simulink model "FlyByWire"  (R2020b)
settings: Solver=FixedStepAuto  StartTime=0.0  StopTime=10.0  FixedStep=0.02  RelTol=1e-3
InitFcn:
  | run('fbw_data_init_fbw_output.m')
values from neighbouring files (symbols this model uses):
  fbw_output_MATLABStruct = struct    [fbw_data_init_fbw_output.m]
undefined symbols (not defined in the file or in its folder): pitch, roll, sim
libraries: fbw_library x19, simulink_extras x13, simulink x2
settings Model: DataDictionary=fbw_data.sldd  Creator=Andreas  LastModifiedBy=Andreas

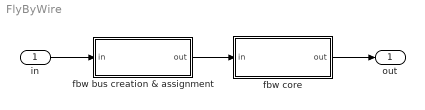
== system FlyByWire ==
  in : Inport  OutDataTypeStr=Bus: fbw_input
  fbw bus creation & assignment : Subsystem
  fbw core : Subsystem
  out : Outport  OutDataTypeStr=Bus: fbw_output
  wires:
  fbw core/1(out) -> out/1
  in/1 -> fbw bus creation & assignment/1(in)
  fbw bus creation & assignment/1(out) -> fbw core/1(in)

== system FlyByWire/fbw bus creation & assignment ==
  in : Inport
  Bus Assignment : BusAssignment  AssignedSignals=sim.raw.time,sim.raw.data,sim.raw.input
  Bus Selector : BusSelector  OutputSignals=time,data,input
  Constant : Constant  Value=fbw_output_MATLABStruct  OutDataTypeStr=Bus: fbw_output
  out : Outport
  wires:
  Constant/1 -> Bus Assignment/1
  in/1 -> Bus Selector/1
  Bus Assignment/1 -> out/1
  Bus Selector/2 -> Bus Assignment/3  "<data>"
  Bus Selector/3 -> Bus Assignment/4  "<input>"
  Bus Selector/1 -> Bus Assignment/2  "<time>"

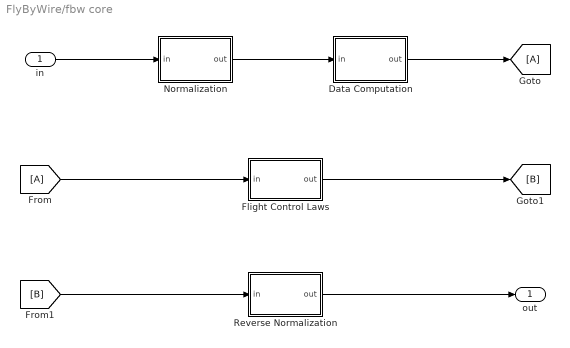
== system FlyByWire/fbw core ==
  in : Inport
  Data Computation : Subsystem
  Flight Control Laws : Subsystem
  Normalization : Subsystem
  Reverse Normalization : Subsystem
  out : Outport
  wires:
  Normalization/1(out) -> Data Computation/1(in)
  [B] -> Reverse Normalization/1(in)
  Data Computation/1(out) -> [A]
  [A] -> Flight Control Laws/1(in)
  in/1 -> Normalization/1(in)
  Reverse Normalization/1(out) -> out/1
  Flight Control Laws/1(out) -> [B]

== system FlyByWire/fbw core/Data Computation ==
  In Bus Element2 : Inport  PortName=in
  In Bus Element1 : Inport  PortName=in
  Bus Assignment : BusAssignment  AssignedSignals=sim.data_computed
  Calculation : Subsystem
  out : Outport
  wires:
  In Bus Element2/1 -> Calculation/1(in)
  In Bus Element1/1 -> Bus Assignment/1
  Bus Assignment/1 -> out/1
  Calculation/1(out) -> Bus Assignment/2

== system FlyByWire/fbw core/Flight Control Laws ==
  In Bus Element3 : Inport  PortName=in
  In Bus Element1 : Inport  PortName=in
  In Bus Element2 : Inport  PortName=in
  Bus Assignment : BusAssignment  AssignedSignals=pitch,roll
  Bus Selector : BusSelector  OutputSignals=roll
  Bus Selector1 : BusSelector  OutputSignals=pitch
  Pitch : Subsystem
  Roll : Subsystem
  out : Outport
  wires:
  Bus Selector1/1 -> Bus Assignment/2  "<pitch>"
  Roll/1(out) -> Bus Selector/1
  In Bus Element1/1 -> Bus Assignment/1
  Bus Selector/1 -> Bus Assignment/3  "<roll>"
  In Bus Element2/1 -> Roll/1(in)
  In Bus Element3/1 -> Pitch/1(in)
  Bus Assignment/1 -> out/1
  Pitch/1(Output) -> Bus Selector1/1

== system FlyByWire/fbw core/Normalization ==
  In Bus Element2 : Inport  PortName=in
  In Bus Element : Inport  PortName=in  Element=sim.raw.data
  In Bus Element1 : Inport  PortName=in  Element=sim.raw.input
  In Bus Element3 : Inport  PortName=in  Element=sim.raw.time
  Bus Assignment : BusAssignment  AssignedSignals=sim.time,sim.data,sim.input
  normalize data : Subsystem
  normalize input : Subsystem
  time : Subsystem
  out : Outport
  wires:
  In Bus Element2/1 -> Bus Assignment/1
  Bus Assignment/1 -> out/1
  In Bus Element/1 -> normalize data/1(in)
  normalize data/1(out) -> Bus Assignment/3
  In Bus Element1/1 -> normalize input/1(in)
  normalize input/1(out) -> Bus Assignment/4
  In Bus Element3/1 -> time/1(in)
  time/1(out) -> Bus Assignment/2

== system FlyByWire/fbw core/Reverse Normalization ==
  In Bus Element9 : Inport  PortName=in
  In Bus Element1 : Inport  PortName=in
  Bus Assignment : BusAssignment  AssignedSignals=sim.raw.output
  Subsystem : Subsystem
  out : Outport
  wires:
  In Bus Element9/1 -> Bus Assignment/1
  Bus Assignment/1 -> out/1
  In Bus Element1/1 -> Subsystem/1(in)
  Subsystem/1(out) -> Bus Assignment/2

== system FlyByWire/fbw core/Data Computation/Calculation ==
  In Bus Element1 : Inport  PortName=in  Element=sim.data.gear_strut_compression_1
  In Bus Element2 : Inport  PortName=in  Element=sim.data.gear_strut_compression_2
  Chart : Stateflow chart  TreatAsAtomicUnit=on
  Out Bus Element : Outport  PortName=out  Element=on_ground
  wires:
  Chart/1(on_ground) -> Out Bus Element/1
  In Bus Element1/1 -> Chart/1(gear_strut_compression_1)
  In Bus Element2/1 -> Chart/2(gear_strut_compression_2)

== system FlyByWire/fbw core/Flight Control Laws/Pitch ==
  in : Inport
  Automatic Trim : Subsystem
  pitch : Subsystem
  pitch:computed : Subsystem
  pitch:integrated : Subsystem
  pitch:output : Subsystem
  pitch:vote : Subsystem
  Output : Outport
  wires:
  Automatic Trim/1(out) -> Output/1
  [A] -> Automatic Trim/1(in)
  pitch:output/1(out) -> [A]
  pitch:integrated/1(out) -> pitch:output/1(in)
  pitch:vote/1(out) -> pitch:integrated/1(in)
  pitch/1(out) -> pitch:vote/1(in)
  in/1 -> pitch:computed/1(in)
  pitch:computed/1(out) -> pitch/1(in)

== system FlyByWire/fbw core/Flight Control Laws/Roll ==
  in : Inport
  roll:computed : Subsystem
  roll:normal : Subsystem
  roll:output : Subsystem
  out : Outport
  wires:
  roll:output/1(out) -> out/1
  roll:normal/1(out) -> roll:output/1(in)
  roll:computed/1(out) -> roll:normal/1(in)
  in/1 -> roll:computed/1(in)

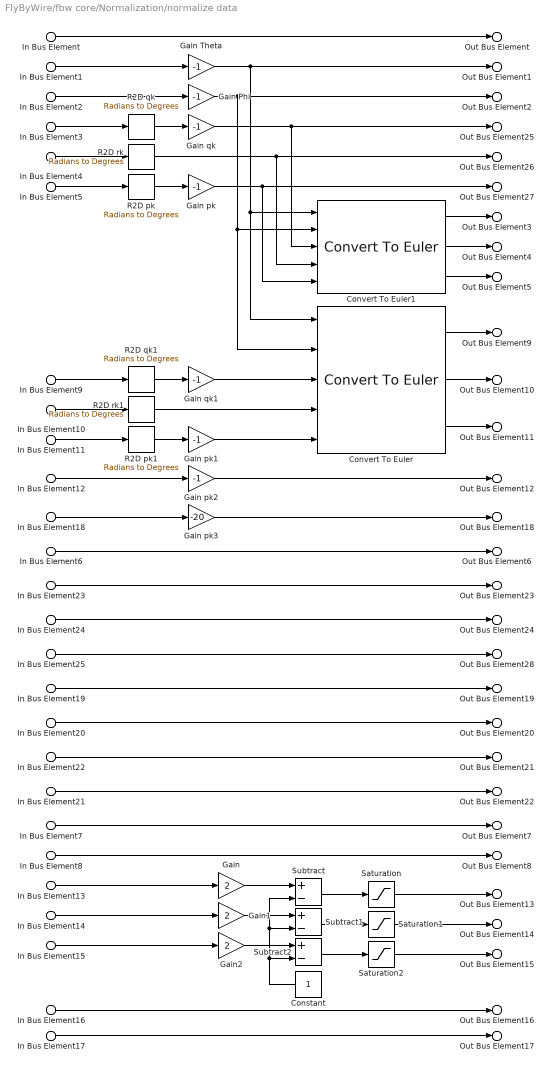
== system FlyByWire/fbw core/Normalization/normalize data ==
  In Bus Element : Inport  PortName=in  Element=nz_g
  In Bus Element1 : Inport  PortName=in  Element=Theta_deg
  In Bus Element2 : Inport  PortName=in  Element=Phi_deg
  In Bus Element3 : Inport  PortName=in  Element=q_rad_s
  In Bus Element4 : Inport  PortName=in  Element=r_rad_s
  In Bus Element5 : Inport  PortName=in  Element=p_rad_s
  In Bus Element6 : Inport  PortName=in  Element=V_ias_kn
  In Bus Element7 : Inport  PortName=in  Element=H_radio_ft
  In Bus Element8 : Inport  PortName=in  Element=CG_percent_MAC
  In Bus Element9 : Inport  PortName=in  Element=q_dot_rad_s2
  In Bus Element10 : Inport  PortName=in  Element=r_dot_rad_s2
  In Bus Element11 : Inport  PortName=in  Element=p_dot_rad_s2
  In Bus Element12 : Inport  PortName=in  Element=eta_trim_deg
  In Bus Element13 : Inport  PortName=in  Element=gear_animation_pos_0
  In Bus Element14 : Inport  PortName=in  Element=gear_animation_pos_1
  In Bus Element15 : Inport  PortName=in  Element=gear_animation_pos_2
  In Bus Element16 : Inport  PortName=in  Element=flaps_handle_index
  In Bus Element17 : Inport  PortName=in  Element=autopilot_master_on
  In Bus Element18 : Inport  PortName=in  Element=zeta_trim_pos
  In Bus Element19 : Inport  PortName=in  Element=V_tas_kn
  In Bus Element20 : Inport  PortName=in  Element=V_mach
  In Bus Element22 : Inport  PortName=in  Element=H_ft
  In Bus Element21 : Inport  PortName=in  Element=H_ind_ft
  In Bus Element23 : Inport  PortName=in  Element=alpha_deg
  In Bus Element24 : Inport  PortName=in  Element=beta_deg
  In Bus Element25 : Inport  PortName=in  Element=beta_dot_deg_s
  Constant : Constant
  Convert To Euler : fbw_library/Convert To Euler  SystemSampleTime=-1  VariantActivationTime=update diagram  Latency=0  AutoFrameSizeCalculation=off
  Convert To Euler1 : fbw_library/Convert To Euler  SystemSampleTime=-1  VariantActivationTime=update diagram  Latency=0  AutoFrameSizeCalculation=off
  Gain : Gain  Gain=2
  Gain Phi : Gain  Gain=-1
  Gain Theta : Gain  Gain=-1
  Gain pk : Gain  Gain=-1
  Gain pk1 : Gain  Gain=-1
  Gain pk2 : Gain  Gain=-1
  Gain pk3 : Gain  Gain=-20
  Gain qk : Gain  Gain=-1
  Gain qk1 : Gain  Gain=-1
  Gain1 : Gain  Gain=2
  Gain2 : Gain  Gain=2
  R2D pk : simulink_extras/Transformations/Radians to Degrees
  R2D pk1 : simulink_extras/Transformations/Radians to Degrees
  R2D qk : simulink_extras/Transformations/Radians to Degrees
  R2D qk1 : simulink_extras/Transformations/Radians to Degrees
  R2D rk : simulink_extras/Transformations/Radians to Degrees
  R2D rk1 : simulink_extras/Transformations/Radians to Degrees
  Saturation : Saturate  UpperLimit=1  LowerLimit=0
  Saturation1 : Saturate  UpperLimit=1  LowerLimit=0
  Saturation2 : Saturate  UpperLimit=1  LowerLimit=0
  Subtract : Sum  Inputs=+-
  Subtract1 : Sum  Inputs=+-
  Subtract2 : Sum  Inputs=+-
  Out Bus Element : Outport  PortName=out  Element=nz_g
  Out Bus Element1 : Outport  PortName=out  Element=Theta_deg
  Out Bus Element2 : Outport  PortName=out  Element=Phi_deg
  Out Bus Element25 : Outport  PortName=out  Element=q_deg_s
  Out Bus Element26 : Outport  PortName=out  Element=r_deg_s
  Out Bus Element27 : Outport  PortName=out  Element=p_deg_s
  Out Bus Element3 : Outport  PortName=out  Element=qk_deg_s
  Out Bus Element4 : Outport  PortName=out  Element=rk_deg_s
  Out Bus Element5 : Outport  PortName=out  Element=pk_deg_s
  Out Bus Element9 : Outport  PortName=out  Element=qk_dot_deg_s2
  Out Bus Element10 : Outport  PortName=out  Element=rk_dot_deg_s2
  Out Bus Element11 : Outport  PortName=out  Element=pk_dot_deg_s2
  Out Bus Element12 : Outport  PortName=out  Element=eta_trim_deg
  Out Bus Element18 : Outport  PortName=out  Element=zeta_trim_deg
  Out Bus Element23 : Outport  PortName=out  Element=alpha_deg
  Out Bus Element24 : Outport  PortName=out  Element=beta_deg
  Out Bus Element28 : Outport  PortName=out  Element=beta_dot_deg_s
  Out Bus Element6 : Outport  PortName=out  Element=V_ias_kn
  Out Bus Element19 : Outport  PortName=out  Element=V_tas_kn
  Out Bus Element20 : Outport  PortName=out  Element=V_mach
  Out Bus Element21 : Outport  PortName=out  Element=H_ft
  Out Bus Element22 : Outport  PortName=out  Element=H_ind_ft
  Out Bus Element7 : Outport  PortName=out  Element=H_radio_ft
  Out Bus Element8 : Outport  PortName=out  Element=CG_percent_MAC
  Out Bus Element13 : Outport  PortName=out  Element=gear_strut_compression_0
  Out Bus Element14 : Outport  PortName=out  Element=gear_strut_compression_1
  Out Bus Element15 : Outport  PortName=out  Element=gear_strut_compression_2
  Out Bus Element16 : Outport  PortName=out  Element=flaps_handle_index
  Out Bus Element17 : Outport  PortName=out  Element=autopilot_master_on
  wires:
  R2D qk/1 -> Gain qk/1
  In Bus Element4/1 -> R2D rk/1
  Gain Phi/1 -> Out Bus Element2/1, Convert To Euler/2, Convert To Euler1/2
  Gain Theta/1 -> Out Bus Element1/1, Convert To Euler/1, Convert To Euler1/1
  In Bus Element7/1 -> Out Bus Element7/1
  In Bus Element2/1 -> Gain Phi/1
  In Bus Element8/1 -> Out Bus Element8/1
  In Bus Element/1 -> Out Bus Element/1
  R2D pk/1 -> Gain pk/1
  In Bus Element6/1 -> Out Bus Element6/1
  In Bus Element1/1 -> Gain Theta/1
  In Bus Element5/1 -> R2D pk/1
  In Bus Element3/1 -> R2D qk/1
  In Bus Element11/1 -> R2D pk1/1
  In Bus Element9/1 -> R2D qk1/1
  R2D qk1/1 -> Gain qk1/1
  R2D pk1/1 -> Gain pk1/1
  In Bus Element10/1 -> R2D rk1/1
  In Bus Element12/1 -> Gain pk2/1
  Gain pk2/1 -> Out Bus Element12/1
  Gain qk1/1 -> Convert To Euler/3
  R2D rk1/1 -> Convert To Euler/4
  Gain pk1/1 -> Convert To Euler/5
  In Bus Element13/1 -> Gain/1
  In Bus Element14/1 -> Gain1/1
  In Bus Element15/1 -> Gain2/1
  Gain/1 -> Subtract/1
  Gain1/1 -> Subtract1/1
  Gain2/1 -> Subtract2/1
  Constant/1 -> Subtract/2, Subtract1/2, Subtract2/2
  Subtract2/1 -> Saturation2/1
  Subtract1/1 -> Saturation1/1
  Subtract/1 -> Saturation/1
  Saturation/1 -> Out Bus Element13/1
  Saturation1/1 -> Out Bus Element14/1
  Saturation2/1 -> Out Bus Element15/1
  In Bus Element16/1 -> Out Bus Element16/1
  In Bus Element17/1 -> Out Bus Element17/1
  In Bus Element18/1 -> Gain pk3/1
  Gain pk3/1 -> Out Bus Element18/1
  In Bus Element19/1 -> Out Bus Element19/1
  In Bus Element20/1 -> Out Bus Element20/1
  In Bus Element22/1 -> Out Bus Element21/1
  In Bus Element21/1 -> Out Bus Element22/1
  In Bus Element23/1 -> Out Bus Element23/1
  In Bus Element24/1 -> Out Bus Element24/1
  Gain qk/1 -> Out Bus Element25/1, Convert To Euler1/3
  R2D rk/1 -> Out Bus Element26/1, Convert To Euler1/4
  Gain pk/1 -> Out Bus Element27/1, Convert To Euler1/5
  Convert To Euler/1 -> Out Bus Element9/1
  Convert To Euler/2 -> Out Bus Element10/1
  Convert To Euler/3 -> Out Bus Element11/1
  Convert To Euler1/1 -> Out Bus Element3/1
  Convert To Euler1/2 -> Out Bus Element4/1
  Convert To Euler1/3 -> Out Bus Element5/1
  In Bus Element25/1 -> Out Bus Element28/1

== system FlyByWire/fbw core/Normalization/normalize input ==
  In Bus Element : Inport  PortName=in  Element=delta_eta_pos
  In Bus Element1 : Inport  PortName=in  Element=delta_xi_pos
  In Bus Element2 : Inport  PortName=in  Element=delta_zeta_pos
  Gain eta : Gain  Gain=-1
  Gain xi : Gain  Gain=-1
  Gain xi1 : Gain  Gain=-1
  Out Bus Element : Outport  PortName=out  Element=delta_eta_pos
  Out Bus Element1 : Outport  PortName=out  Element=delta_xi_pos
  Out Bus Element2 : Outport  PortName=out  Element=delta_zeta_pos
  wires:
  In Bus Element/1 -> Gain eta/1
  Gain xi/1 -> Out Bus Element1/1
  Gain eta/1 -> Out Bus Element/1
  In Bus Element1/1 -> Gain xi/1
  In Bus Element2/1 -> Gain xi1/1
  Gain xi1/1 -> Out Bus Element2/1

== system FlyByWire/fbw core/Normalization/time ==
  In Bus Element : Inport  PortName=in  Element=dt
  Delay : Delay  DelayLength=1
  Sum : Sum  Inputs=|++
  Out Bus Element : Outport  PortName=out  Element=dt
  Out Bus Element1 : Outport  PortName=out  Element=monotonic_time
  wires:
  Sum/1 -> Delay/1, Out Bus Element1/1
  In Bus Element/1 -> Sum/1, Out Bus Element/1
  Delay/1 -> Sum/2

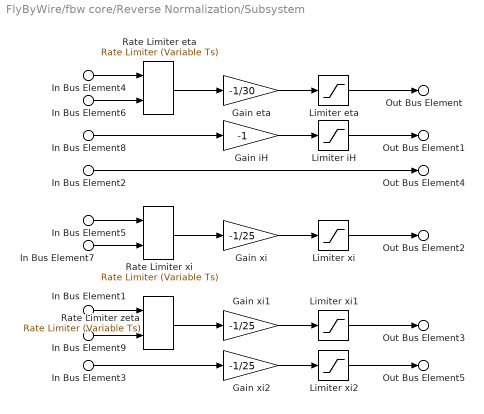
== system FlyByWire/fbw core/Reverse Normalization/Subsystem ==
  In Bus Element4 : Inport  PortName=in  Element=pitch.output.eta_deg
  In Bus Element8 : Inport  PortName=in  Element=pitch.output.eta_trim_deg
  In Bus Element2 : Inport  PortName=in  Element=pitch.data_computed.eta_trim_deg_should_write
  In Bus Element5 : Inport  PortName=in  Element=roll.output.xi_deg
  In Bus Element1 : Inport  PortName=in  Element=roll.output.zeta_deg
  In Bus Element3 : Inport  PortName=in  Element=sim.data.zeta_trim_deg
  In Bus Element6 : Inport  PortName=in  Element=sim.time.dt
  In Bus Element7 : Inport  PortName=in  Element=sim.time.dt
  In Bus Element9 : Inport  PortName=in  Element=sim.time.dt
  Gain eta : Gain  Gain=-1/30
  Gain iH : Gain  Gain=-1
  Gain xi : Gain  Gain=-1/25
  Gain xi1 : Gain  Gain=-1/25
  Gain xi2 : Gain  Gain=-1/25
  Limiter eta : Saturate  UpperLimit=1.0  LowerLimit=-1.0
  Limiter iH : Saturate  UpperLimit=13  LowerLimit=-3.5
  Limiter xi : Saturate  UpperLimit=1.0  LowerLimit=-1.0
  Limiter xi1 : Saturate  UpperLimit=1.0  LowerLimit=-1.0
  Limiter xi2 : Saturate  UpperLimit=1.0  LowerLimit=-1.0
  Rate Limiter eta : fbw_library/Rate Limiter (Variable Ts)  up=45  lo=-45  InitialCondition=0.0
  Rate Limiter xi : fbw_library/Rate Limiter (Variable Ts)  up=50  lo=-50  InitialCondition=0.0
  Rate Limiter zeta : fbw_library/Rate Limiter (Variable Ts)  up=45  lo=-45  InitialCondition=0.0
  Out Bus Element : Outport  PortName=out  Element=eta_pos
  Out Bus Element1 : Outport  PortName=out  Element=eta_trim_deg
  Out Bus Element4 : Outport  PortName=out  Element=eta_trim_deg_should_write
  Out Bus Element2 : Outport  PortName=out  Element=xi_pos
  Out Bus Element3 : Outport  PortName=out  Element=zeta_pos
  Out Bus Element5 : Outport  PortName=out  Element=zeta_trim_pos
  wires:
  Gain xi/1 -> Limiter xi/1
  Rate Limiter xi/1 -> Gain xi/1
  Rate Limiter eta/1 -> Gain eta/1
  Limiter iH/1 -> Out Bus Element1/1
  Gain eta/1 -> Limiter eta/1
  Gain iH/1 -> Limiter iH/1
  Limiter eta/1 -> Out Bus Element/1
  Limiter xi/1 -> Out Bus Element2/1
  In Bus Element4/1 -> Rate Limiter eta/1
  In Bus Element8/1 -> Gain iH/1
  In Bus Element5/1 -> Rate Limiter xi/1
  Rate Limiter zeta/1 -> Gain xi1/1
  Limiter xi1/1 -> Out Bus Element3/1
  In Bus Element1/1 -> Rate Limiter zeta/1
  Gain xi1/1 -> Limiter xi1/1
  In Bus Element2/1 -> Out Bus Element4/1
  In Bus Element3/1 -> Gain xi2/1
  Gain xi2/1 -> Limiter xi2/1
  Limiter xi2/1 -> Out Bus Element5/1
  In Bus Element6/1 -> Rate Limiter eta/2
  In Bus Element7/1 -> Rate Limiter xi/2
  In Bus Element9/1 -> Rate Limiter zeta/2

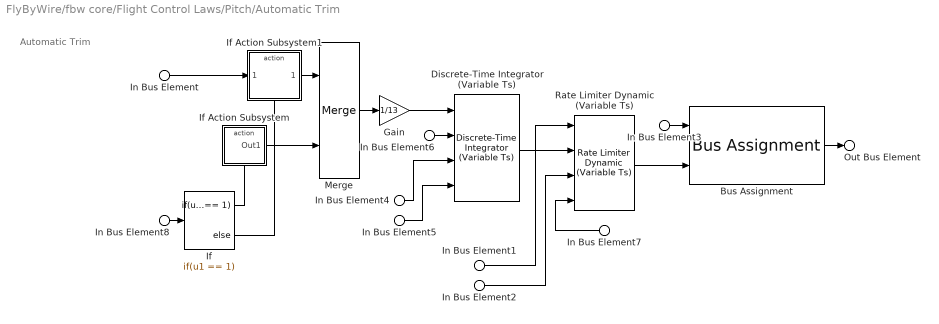
== system FlyByWire/fbw core/Flight Control Laws/Pitch/Automatic Trim ==
  note: Automatic Trim
  In Bus Element3 : Inport  PortName=in
  In Bus Element : Inport  PortName=in  Element=pitch.integrated.eta_deg
  In Bus Element8 : Inport  PortName=in  Element=pitch.data_computed.eta_trim_deg_should_freeze
  In Bus Element5 : Inport  PortName=in  Element=pitch.data_computed.eta_trim_deg_reset_deg
  In Bus Element4 : Inport  PortName=in  Element=pitch.data_computed.eta_trim_deg_reset
  In Bus Element1 : Inport  PortName=in  Element=pitch.data_computed.eta_trim_deg_rate_limit_up_deg_s
  In Bus Element2 : Inport  PortName=in  Element=pitch.data_computed.eta_trim_deg_rate_limit_lo_deg_s
  In Bus Element6 : Inport  PortName=in  Element=sim.time.dt
  In Bus Element7 : Inport  PortName=in  Element=sim.time.dt
  Bus Assignment : BusAssignment  AssignedSignals=pitch.output.eta_trim_deg
  Discrete-Time Integrator (Variable Ts) : fbw_library/Discrete-Time Integrator (Variable Ts)  Gain=1.0  ExternalReset=Level  InitialConditionSource=Input port  InitialCondition=0.0  UpperLimit=3.5  LowerLimit=-11
  Gain : Gain  Gain=1/13
  If : If  IfExpression=u1 == 1
  If Action Subsystem : Subsystem  TreatAsAtomicUnit=on
  If Action Subsystem1 : Subsystem  TreatAsAtomicUnit=on
  Merge : Merge
  Rate Limiter Dynamic (Variable Ts) : fbw_library/Rate Limiter Dynamic (Variable Ts)  InitialCondition=0.0
  Out Bus Element : Outport  PortName=out
  wires:
  In Bus Element3/1 -> Bus Assignment/1
  If Action Subsystem/1(Out1) -> Merge/2
  Discrete-Time Integrator (Variable Ts)/1 -> Rate Limiter Dynamic (Variable Ts)/2
  If Action Subsystem1/1(Out1) -> Merge/1
  Merge/1 -> Gain/1
  If/1 -> If Action Subsystem/Action
  If/2 -> If Action Subsystem1/Action
  In Bus Element/1 -> If Action Subsystem1/1(η (°))
  Bus Assignment/1 -> Out Bus Element/1
  In Bus Element1/1 -> Rate Limiter Dynamic (Variable Ts)/1
  In Bus Element2/1 -> Rate Limiter Dynamic (Variable Ts)/3
  In Bus Element5/1 -> Discrete-Time Integrator (Variable Ts)/4
  Gain/1 -> Discrete-Time Integrator (Variable Ts)/1
  Rate Limiter Dynamic (Variable Ts)/1 -> Bus Assignment/2
  In Bus Element8/1 -> If/1
  In Bus Element4/1 -> Discrete-Time Integrator (Variable Ts)/3
  In Bus Element6/1 -> Discrete-Time Integrator (Variable Ts)/2
  In Bus Element7/1 -> Rate Limiter Dynamic (Variable Ts)/4

== system FlyByWire/fbw core/Flight Control Laws/Pitch/pitch ==
  note: Pitch Laws
  In Bus Element2 : Inport  PortName=in
  In Bus Element5 : Inport  PortName=in
  Bus Assignment : BusAssignment  AssignedSignals=pitch.law_normal
  Bus Selector1 : BusSelector  OutputSignals=pitch.law_normal
  law_normal : Subsystem
  Out Bus Element3 : Outport  PortName=out
  wires:
  Bus Selector1/1 -> Bus Assignment/2  "<law_normal>"
  In Bus Element2/1 -> law_normal/1(in)
  In Bus Element5/1 -> Bus Assignment/1
  Bus Assignment/1 -> Out Bus Element3/1
  law_normal/1(out) -> Bus Selector1/1

== system FlyByWire/fbw core/Flight Control Laws/Pitch/pitch:computed ==
  In Bus Element3 : Inport  PortName=in
  In Bus Element1 : Inport  PortName=in
  Bus Assignment : BusAssignment  AssignedSignals=pitch.data_computed
  computation : Subsystem
  Out Bus Element1 : Outport  PortName=out
  wires:
  computation/1(out) -> Bus Assignment/2
  In Bus Element3/1 -> computation/1(in)
  In Bus Element1/1 -> Bus Assignment/1
  Bus Assignment/1 -> Out Bus Element1/1

== system FlyByWire/fbw core/Flight Control Laws/Pitch/pitch:integrated ==
  note: Integration
  In Bus Element : Inport  PortName=in
  In Bus Element8 : Inport  PortName=in  Element=pitch.vote.eta_dot_deg_s
  In Bus Element11 : Inport  PortName=in  Element=pitch.data_computed.in_flight
  In Bus Element9 : Inport  PortName=in  Element=pitch.data_computed.delta_eta_deg
  In Bus Element1 : Inport  PortName=in  Element=sim.time.dt
  Bus Assignment : BusAssignment  AssignedSignals=pitch.integrated.eta_deg
  Discrete-Time Integrator (Variable Ts) : fbw_library/Discrete-Time Integrator (Variable Ts)  Gain=1.0  ExternalReset=Rising  InitialConditionSource=Input port  InitialCondition=0.0  UpperLimit=17  LowerLimit=-30
  Out Bus Element : Outport  PortName=out
  wires:
  In Bus Element8/1 -> Discrete-Time Integrator (Variable Ts)/1
  In Bus Element11/1 -> Discrete-Time Integrator (Variable Ts)/3
  In Bus Element/1 -> Bus Assignment/1
  Bus Assignment/1 -> Out Bus Element/1
  Discrete-Time Integrator (Variable Ts)/1 -> Bus Assignment/2
  In Bus Element9/1 -> Discrete-Time Integrator (Variable Ts)/4
  In Bus Element1/1 -> Discrete-Time Integrator (Variable Ts)/2

== system FlyByWire/fbw core/Flight Control Laws/Pitch/pitch:output ==
  In Bus Element : Inport  PortName=in
  In Bus Element1 : Inport  PortName=in  Element=pitch.integrated.eta_deg
  In Bus Element3 : Inport  PortName=in  Element=pitch.data_computed.in_flight_gain
  In Bus Element2 : Inport  PortName=in  Element=pitch.data_computed.delta_eta_deg
  Bus Assignment : BusAssignment  AssignedSignals=pitch.output.eta_deg
  Signal Blending : fbw_library/Signal Blending  SystemSampleTime=-1  VariantActivationTime=update diagram  Latency=0  AutoFrameSizeCalculation=off
  Out Bus Element : Outport  PortName=out
  wires:
  Signal Blending/1 -> Bus Assignment/2
  In Bus Element3/1 -> Signal Blending/3
  In Bus Element1/1 -> Signal Blending/1
  In Bus Element/1 -> Bus Assignment/1
  Bus Assignment/1 -> Out Bus Element/1
  In Bus Element2/1 -> Signal Blending/2

== system FlyByWire/fbw core/Flight Control Laws/Pitch/pitch:vote ==
  note: Voting of active law
  In Bus Element1 : Inport  PortName=in
  Bus Element In : Inport  PortName=in  Element=pitch.law_normal.eta_dot_deg_s
  Bus Assignment : BusAssignment  AssignedSignals=pitch.vote.eta_dot_deg_s
  Mux : Mux  Inputs=1
  Voter : MATLAB Function  TreatAsAtomicUnit=on
  Out Bus Element1 : Outport  PortName=out
  wires:
  Bus Element In/1 -> Mux/1
  In Bus Element1/1 -> Bus Assignment/1
  Bus Assignment/1 -> Out Bus Element1/1
  Voter/1(vote) -> Bus Assignment/2
  Mux/1 -> Voter/1(input)

== system FlyByWire/fbw core/Flight Control Laws/Roll/roll:computed ==
  In Bus Element3 : Inport  PortName=in
  In Bus Element1 : Inport  PortName=in
  Bus Assignment : BusAssignment  AssignedSignals=roll.data_computed
  computation : Subsystem
  Out Bus Element1 : Outport  PortName=out
  wires:
  computation/1(out) -> Bus Assignment/2
  In Bus Element3/1 -> computation/1(in)
  In Bus Element1/1 -> Bus Assignment/1
  Bus Assignment/1 -> Out Bus Element1/1

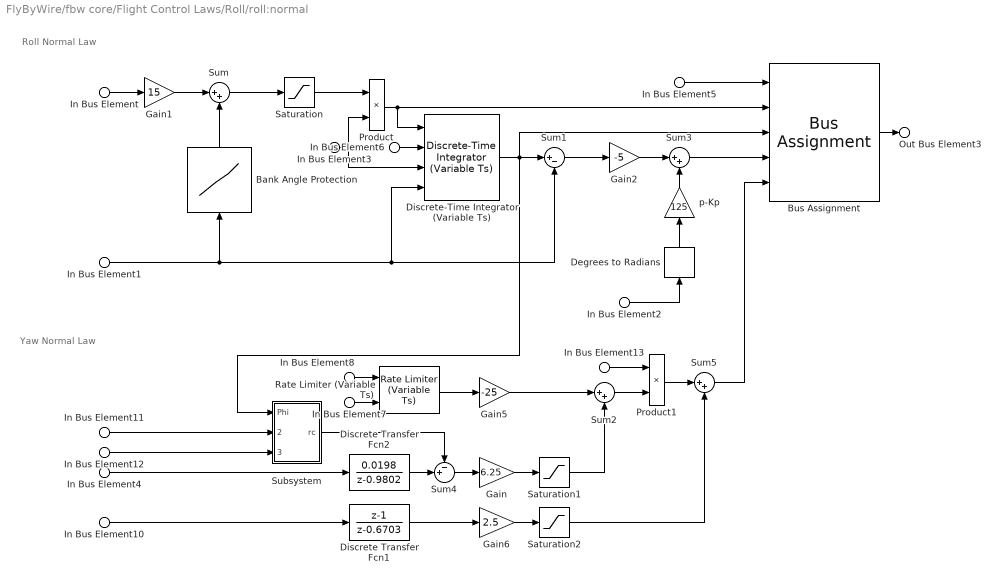
== system FlyByWire/fbw core/Flight Control Laws/Roll/roll:normal ==
  note: Yaw Normal Law
  note: Roll Normal Law
  In Bus Element5 : Inport  PortName=in
  In Bus Element : Inport  PortName=in  Element=sim.input.delta_xi_pos
  In Bus Element8 : Inport  PortName=in  Element=sim.input.delta_zeta_pos
  In Bus Element1 : Inport  PortName=in  Element=sim.data.Phi_deg
  In Bus Element2 : Inport  PortName=in  Element=sim.data.pk_deg_s
  In Bus Element10 : Inport  PortName=in  Element=sim.data.r_deg_s
  In Bus Element4 : Inport  PortName=in  Element=sim.data.r_deg_s
  In Bus Element11 : Inport  PortName=in  Element=sim.data.Theta_deg
  In Bus Element12 : Inport  PortName=in  Element=sim.data.V_tas_kn
  In Bus Element6 : Inport  PortName=in  Element=sim.time.dt
  In Bus Element7 : Inport  PortName=in  Element=sim.time.dt
  In Bus Element3 : Inport  PortName=in  Element=roll.data_computed.in_flight_gain
  In Bus Element13 : Inport  PortName=in  Element=roll.data_computed.in_flight_gain
  Bank Angle Protection : Lookup_n-D  NumberOfTableDimensions=1  BreakpointsForDimension1=[-90,-66,-33,0,33,66,90]  Table=[15,15,0,0,0,-15,-15]  InternalRulePriority=Speed  RndMeth=Simplest  InputSameDT=on
  Bus Assignment : BusAssignment  AssignedSignals=roll.law_normal.pk_c_deg_s,roll.law_normal.Phi_c_deg,roll.law_normal.xi_deg,roll.law_normal.zeta_deg
  Degrees to Radians : simulink_extras/Transformations/Degrees to Radians
  Discrete Transfer Fcn1 : DiscreteTransferFcn  Numerator=[1 -1]  Denominator=[1 -0.6703]
  Discrete Transfer Fcn2 : DiscreteTransferFcn  Numerator=[0.0198]  Denominator=[1 -0.9802]
  Discrete-Time Integrator (Variable Ts) : fbw_library/Discrete-Time Integrator (Variable Ts)  Gain=1.0  ExternalReset=Rising  InitialConditionSource=Input port  InitialCondition=0.0  UpperLimit=67  LowerLimit=-67
  Gain : Gain  Gain=6.25
  Gain1 : Gain  Gain=15
  Gain2 : Gain  Gain=-5
  Gain5 : Gain  Gain=-25
  Gain6 : Gain  Gain=2.5
  Product : Product
  Product1 : Product
  Rate Limiter (Variable Ts) : fbw_library/Rate Limiter (Variable Ts)  up=1.0  lo=-1.0  InitialCondition=0.0
  Saturation : Saturate  UpperLimit=15  LowerLimit=-15
  Saturation1 : Saturate  UpperLimit=25  LowerLimit=-25
  Saturation2 : Saturate  UpperLimit=25  LowerLimit=-25
  Subsystem : Subsystem
      mask Display:
      | port_label('input', 1, '\Phi', 'texmode', 'on');
      | port_label('input', 2, '\Theta', 'texmode', 'on');
      | port_label('input', 3, 'V_{TAS}', 'texmode', 'on');
      | 
      | port_label('output', 1, 'r_c', 'texmode', 'on');
  Sum{,2..3,5} (4 alike) : Sum  Inputs=|++
  Sum1 : Sum  Inputs=|+-
  Sum4 : Sum  Inputs=-+|
  p-Kp : Gain  Gain=125
  Out Bus Element3 : Outport  PortName=out
  wires:
  In Bus Element5/1 -> Bus Assignment/1
  In Bus Element2/1 -> Degrees to Radians/1
  In Bus Element1/1 -> Bank Angle Protection/1, Sum1/2, Discrete-Time Integrator (Variable Ts)/4
  In Bus Element/1 -> Gain1/1
  Product/1 -> Bus Assignment/2, Discrete-Time Integrator (Variable Ts)/1
  Saturation/1 -> Product/1
  In Bus Element3/1 -> Discrete-Time Integrator (Variable Ts)/3, Product/2
  Discrete-Time Integrator (Variable Ts)/1 -> Bus Assignment/3, Sum1/1, Subsystem/1(Phi)
  Degrees to Radians/1 -> p-Kp/1
  Gain1/1 -> Sum/1
  Sum1/1 -> Gain2/1
  Gain2/1 -> Sum3/1
  p-Kp/1 -> Sum3/2
  Bank Angle Protection/1 -> Sum/2
  Sum/1 -> Saturation/1
  Bus Assignment/1 -> Out Bus Element3/1
  Sum2/1 -> Product1/2
  Gain/1 -> Saturation1/1
  In Bus Element10/1 -> Discrete Transfer Fcn1/1
  Saturation1/1 -> Sum2/2
  In Bus Element8/1 -> Rate Limiter (Variable Ts)/1
  Gain5/1 -> Sum2/1
  In Bus Element11/1 -> Subsystem/2(Theta)
  In Bus Element12/1 -> Subsystem/3(V_tas)
  Subsystem/1(rc) -> Sum4/1
  Discrete Transfer Fcn1/1 -> Gain6/1
  Gain6/1 -> Saturation2/1
  Saturation2/1 -> Sum5/2
  Sum4/1 -> Gain/1
  Discrete Transfer Fcn2/1 -> Sum4/2
  Rate Limiter (Variable Ts)/1 -> Gain5/1
  Sum5/1 -> Bus Assignment/5
  Product1/1 -> Sum5/1
  In Bus Element13/1 -> Product1/1
  Sum3/1 -> Bus Assignment/4
  In Bus Element4/1 -> Discrete Transfer Fcn2/1
  In Bus Element6/1 -> Discrete-Time Integrator (Variable Ts)/2
  In Bus Element7/1 -> Rate Limiter (Variable Ts)/2

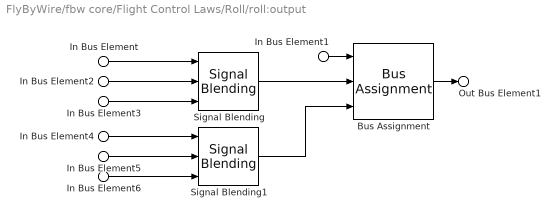
== system FlyByWire/fbw core/Flight Control Laws/Roll/roll:output ==
  In Bus Element1 : Inport  PortName=in
  In Bus Element : Inport  PortName=in  Element=roll.law_normal.xi_deg
  In Bus Element4 : Inport  PortName=in  Element=roll.law_normal.zeta_deg
  In Bus Element3 : Inport  PortName=in  Element=roll.data_computed.in_flight_gain
  In Bus Element6 : Inport  PortName=in  Element=roll.data_computed.in_flight_gain
  In Bus Element2 : Inport  PortName=in  Element=roll.data_computed.delta_xi_deg
  In Bus Element5 : Inport  PortName=in  Element=roll.data_computed.delta_zeta_deg
  Bus Assignment : BusAssignment  AssignedSignals=roll.output.xi_deg,roll.output.zeta_deg
  Signal Blending : fbw_library/Signal Blending  SystemSampleTime=-1  VariantActivationTime=update diagram  Latency=0  AutoFrameSizeCalculation=off
  Signal Blending1 : fbw_library/Signal Blending  SystemSampleTime=-1  VariantActivationTime=update diagram  Latency=0  AutoFrameSizeCalculation=off
  Out Bus Element1 : Outport  PortName=out
  wires:
  Signal Blending/1 -> Bus Assignment/2
  In Bus Element3/1 -> Signal Blending/3
  In Bus Element/1 -> Signal Blending/1
  In Bus Element1/1 -> Bus Assignment/1
  Bus Assignment/1 -> Out Bus Element1/1
  In Bus Element4/1 -> Signal Blending1/1
  In Bus Element6/1 -> Signal Blending1/3
  Signal Blending1/1 -> Bus Assignment/3
  In Bus Element2/1 -> Signal Blending/2
  In Bus Element5/1 -> Signal Blending1/2

== system FlyByWire/fbw core/Flight Control Laws/Pitch/Automatic Trim/If Action Subsystem ==
  Action Port : ActionPort  InitializeStates=reset  ActionPortLabel=if(u1 == 1)
  Constant : Constant  Value=0
  Out1 : Outport
  wires:
  Constant/1 -> Out1/1

== system FlyByWire/fbw core/Flight Control Laws/Pitch/Automatic Trim/If Action Subsystem1 ==
  η (°) : Inport
  Action Port : ActionPort  ActionPortLabel=else
  Out1 : Outport
  wires:
  η (°)/1 -> Out1/1

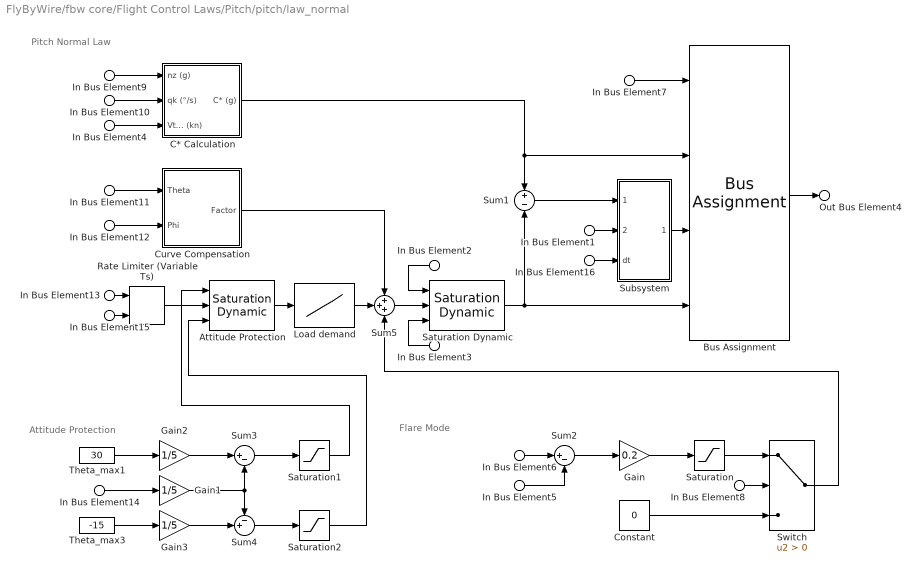
== system FlyByWire/fbw core/Flight Control Laws/Pitch/pitch/law_normal ==
  note: Attitude Protection
  note: Flare Mode
  note: Pitch Normal Law
  In Bus Element7 : Inport  PortName=in
  In Bus Element9 : Inport  PortName=in  Element=sim.data.nz_g
  In Bus Element11 : Inport  PortName=in  Element=sim.data.Theta_deg
  In Bus Element5 : Inport  PortName=in  Element=sim.data.Theta_deg
  In Bus Element14 : Inport  PortName=in  Element=sim.data.Theta_deg
  In Bus Element12 : Inport  PortName=in  Element=sim.data.Phi_deg
  In Bus Element10 : Inport  PortName=in  Element=sim.data.qk_deg_s
  In Bus Element1 : Inport  PortName=in  Element=sim.data.V_tas_kn
  In Bus Element4 : Inport  PortName=in  Element=sim.data.V_tas_kn
  In Bus Element13 : Inport  PortName=in  Element=sim.input.delta_eta_pos
  In Bus Element15 : Inport  PortName=in  Element=sim.time.dt
  In Bus Element16 : Inport  PortName=in  Element=sim.time.dt
  In Bus Element2 : Inport  PortName=in  Element=pitch.data_computed.nz_limit_up_g
  In Bus Element3 : Inport  PortName=in  Element=pitch.data_computed.nz_limit_lo_g
  In Bus Element6 : Inport  PortName=in  Element=pitch.data_computed.flare_Theta_c_deg
  In Bus Element8 : Inport  PortName=in  Element=pitch.data_computed.in_flare
  Attitude Protection : simulink/Discontinuities/Saturation Dynamic  OutMin=[]  OutMax=[]  OutDataTypeStr=Inherit: Same as second input  OutDataType=fixdt(1, 16)  OutScaling=2^-10  DoSatur=off
  Bus Assignment : BusAssignment  AssignedSignals=pitch.law_normal.Cstar_g,pitch.law_normal.eta_dot_deg_s,pitch.law_normal.nz_c_g
  C* Calculation : Subsystem
      mask Display:
      | disp('')
      | port_label('input', 1, 'n_z [g]','interpreter','tex')
      | port_label('input', 2, 'q [°/s]','interpreter','tex')
      | port_label('output', 1, 'C* [g]','interpreter','tex')
  Constant : Constant  Value=0
  Curve Compensation : Subsystem
      mask Display:
      | disp('')
      | port_label('input', 1, '\Theta [°]','interpreter','tex')
      | port_label('input', 2, '\Phi [°]','interpreter','tex')
      | port_label('output', 1, 'Factor','interpreter','tex')
  Gain : Gain  Gain=0.2
  Gain1 : Gain  Gain=1/5
  Gain2 : Gain  Gain=1/5
  Gain3 : Gain  Gain=1/5
  Load demand : Lookup_n-D  NumberOfTableDimensions=1  BreakpointsForDimension1=[-1 0 1]  Table=[-2 0 1.5]  InternalRulePriority=Speed  RndMeth=Simplest  InputSameDT=on
  Rate Limiter (Variable Ts) : fbw_library/Rate Limiter (Variable Ts)  up=1.0  lo=-1.0  InitialCondition=0.0
  Saturation : Saturate  UpperLimit=0  LowerLimit=-0.6
  Saturation Dynamic : simulink/Discontinuities/Saturation Dynamic  OutMin=[]  OutMax=[]  OutDataTypeStr=Inherit: Same as second input  OutDataType=fixdt(1, 16)  OutScaling=2^-10  DoSatur=off
  Saturation1 : Saturate  UpperLimit=1  LowerLimit=-0.25
  Saturation2 : Saturate  UpperLimit=0.25  LowerLimit=-1
  Subsystem : Subsystem
      mask Display:
      | port_label('input', 1, 'C* error', 'texmode', 'on')
      | port_label('input', 2, 'V_k', 'texmode', 'on')
      | 
      | port_label('output', 1, '\eta dot', 'texmode', 'on')
  Sum1 : Sum  Inputs=+-
  Sum2 : Sum  Inputs=|+-
  Sum3 : Sum  Inputs=|+-
  Sum4 : Sum  Inputs=-+|
  Sum5 : Sum  Inputs=+++
  Switch : Switch  Criteria=u2 > Threshold
  Theta_max1 : Constant  Value=30
  Theta_max3 : Constant  Value=-15
  Out Bus Element4 : Outport  PortName=out
  wires:
  In Bus Element7/1 -> Bus Assignment/1
  In Bus Element12/1 -> Curve Compensation/2(Phi)
  In Bus Element11/1 -> Curve Compensation/1(Theta)
  C* Calculation/1(C* (g)) -> Sum1/1, Bus Assignment/2
  Curve Compensation/1(Factor) -> Sum5/1
  Bus Assignment/1 -> Out Bus Element4/1
  Sum1/1 -> Subsystem/1(delta_cstar_g)
  In Bus Element1/1 -> Subsystem/2(Vk_kt)
  Subsystem/1(eta_dot_deg_s) -> Bus Assignment/3
  In Bus Element2/1 -> Saturation Dynamic/1
  In Bus Element3/1 -> Saturation Dynamic/3
  In Bus Element4/1 -> C* Calculation/3(Vtas (kn))
  In Bus Element9/1 -> C* Calculation/1(nz (g))
  In Bus Element10/1 -> C* Calculation/2(qk (°/s))
  In Bus Element5/1 -> Sum2/2
  Sum2/1 -> Gain/1
  In Bus Element6/1 -> Sum2/1
  Gain/1 -> Saturation/1
  In Bus Element8/1 -> Switch/2
  Constant/1 -> Switch/3
  Switch/1 -> Sum5/3
  Saturation Dynamic/1 -> Bus Assignment/4, Sum1/2
  Sum5/1 -> Saturation Dynamic/2
  Saturation/1 -> Switch/1
  In Bus Element13/1 -> Rate Limiter (Variable Ts)/1
  In Bus Element14/1 -> Gain1/1
  Theta_max1/1 -> Gain2/1
  Gain2/1 -> Sum3/1
  Gain1/1 -> Sum4/1, Sum3/2
  Theta_max3/1 -> Gain3/1
  Gain3/1 -> Sum4/2
  Sum3/1 -> Saturation1/1
  Sum4/1 -> Saturation2/1
  Saturation1/1 -> Attitude Protection/1
  Saturation2/1 -> Attitude Protection/3
  Attitude Protection/1 -> Load demand/1
  Load demand/1 -> Sum5/2
  Rate Limiter (Variable Ts)/1 -> Attitude Protection/2
  In Bus Element15/1 -> Rate Limiter (Variable Ts)/2
  In Bus Element16/1 -> Subsystem/3(dt)

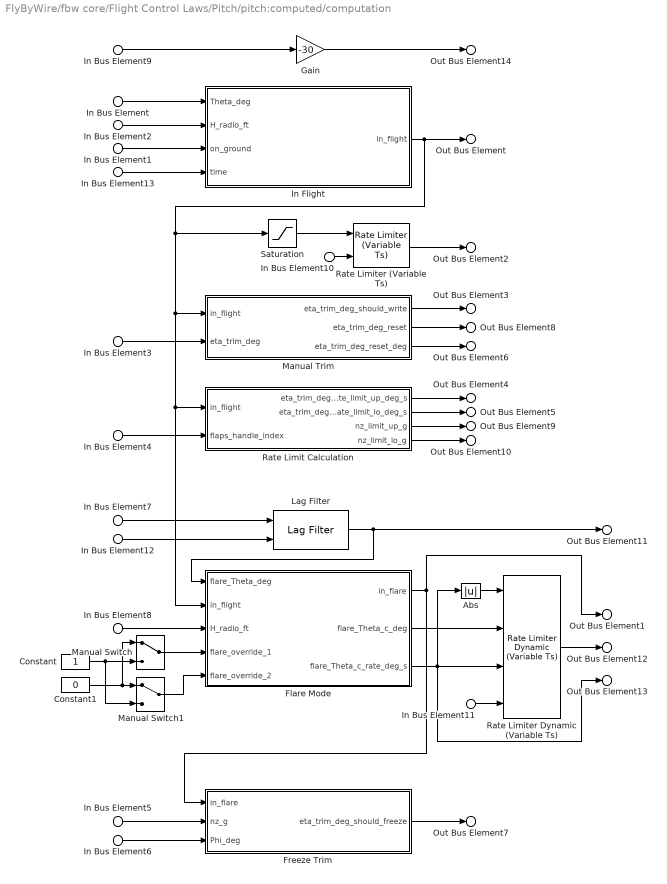
== system FlyByWire/fbw core/Flight Control Laws/Pitch/pitch:computed/computation ==
  In Bus Element : Inport  PortName=in  Element=sim.data.Theta_deg
  In Bus Element7 : Inport  PortName=in  Element=sim.data.Theta_deg
  In Bus Element2 : Inport  PortName=in  Element=sim.data.H_radio_ft
  In Bus Element8 : Inport  PortName=in  Element=sim.data.H_radio_ft
  In Bus Element3 : Inport  PortName=in  Element=sim.data.eta_trim_deg
  In Bus Element4 : Inport  PortName=in  Element=sim.data.flaps_handle_index
  In Bus Element5 : Inport  PortName=in  Element=sim.data.nz_g
  In Bus Element6 : Inport  PortName=in  Element=sim.data.Phi_deg
  In Bus Element1 : Inport  PortName=in  Element=sim.data_computed.on_ground
  In Bus Element9 : Inport  PortName=in  Element=sim.input.delta_eta_pos
  In Bus Element10 : Inport  PortName=in  Element=sim.time.dt
  In Bus Element11 : Inport  PortName=in  Element=sim.time.dt
  In Bus Element12 : Inport  PortName=in  Element=sim.time.dt
  In Bus Element13 : Inport  PortName=in  Element=sim.time.monotonic_time
  Abs : Abs
  Constant : Constant
  Constant1 : Constant  Value=0
  Flare Mode : Stateflow chart  TreatAsAtomicUnit=on
  Freeze Trim : Stateflow chart  TreatAsAtomicUnit=on
  Gain : Gain  Gain=-30
  In Flight : Stateflow chart  TreatAsAtomicUnit=on
  Lag Filter : fbw_library/Lag Filter  C1=1/20
  Manual Switch : ManualSwitch
  Manual Switch1 : ManualSwitch
  Manual Trim : Stateflow chart  TreatAsAtomicUnit=on
  Rate Limit Calculation : Stateflow chart  TreatAsAtomicUnit=on
  Rate Limiter (Variable Ts) : fbw_library/Rate Limiter (Variable Ts)  up=1/5  lo=-1/5  InitialCondition=0.0
  Rate Limiter Dynamic (Variable Ts) : fbw_library/Rate Limiter Dynamic (Variable Ts)  InitialCondition=0.0
  Saturation : Saturate  UpperLimit=1  LowerLimit=0
  Out Bus Element14 : Outport  PortName=out  Element=delta_eta_deg
  Out Bus Element : Outport  PortName=out  Element=in_flight
  Out Bus Element1 : Outport  PortName=out  Element=in_flare
  Out Bus Element2 : Outport  PortName=out  Element=in_flight_gain
  Out Bus Element9 : Outport  PortName=out  Element=nz_limit_up_g
  Out Bus Element10 : Outport  PortName=out  Element=nz_limit_lo_g
  Out Bus Element7 : Outport  PortName=out  Element=eta_trim_deg_should_freeze
  Out Bus Element8 : Outport  PortName=out  Element=eta_trim_deg_reset
  Out Bus Element6 : Outport  PortName=out  Element=eta_trim_deg_reset_deg
  Out Bus Element3 : Outport  PortName=out  Element=eta_trim_deg_should_write
  Out Bus Element4 : Outport  PortName=out  Element=eta_trim_deg_rate_limit_up_deg_s
  Out Bus Element5 : Outport  PortName=out  Element=eta_trim_deg_rate_limit_lo_deg_s
  Out Bus Element11 : Outport  PortName=out  Element=flare_Theta_deg
  Out Bus Element12 : Outport  PortName=out  Element=flare_Theta_c_deg
  Out Bus Element13 : Outport  PortName=out  Element=flare_Theta_c_rate_deg_s
  wires:
  Saturation/1 -> Rate Limiter (Variable Ts)/1
  In Flight/1(in_flight) -> Flare Mode/2(in_flight), Rate Limit Calculation/1(in_flight), Manual Trim/1(in_flight), Saturation/1, Out Bus Element/1
  In Bus Element1/1 -> In Flight/3(on_ground)
  In Bus Element2/1 -> In Flight/2(H_radio_ft)
  In Bus Element/1 -> In Flight/1(Theta_deg)
  Manual Trim/1(eta_trim_deg_should_write) -> Out Bus Element3/1
  In Bus Element3/1 -> Manual Trim/2(eta_trim_deg)
  Manual Trim/3(eta_trim_deg_reset_deg) -> Out Bus Element6/1
  Rate Limit Calculation/1(eta_trim_deg_rate_limit_up_deg_s) -> Out Bus Element4/1
  Rate Limit Calculation/2(eta_trim_deg_rate_limit_lo_deg_s) -> Out Bus Element5/1
  In Bus Element4/1 -> Rate Limit Calculation/2(flaps_handle_index)
  Freeze Trim/1(eta_trim_deg_should_freeze) -> Out Bus Element7/1
  In Bus Element6/1 -> Freeze Trim/3(Phi_deg)
  In Bus Element5/1 -> Freeze Trim/2(nz_g)
  Manual Trim/2(eta_trim_deg_reset) -> Out Bus Element8/1
  Rate Limit Calculation/3(nz_limit_up_g) -> Out Bus Element9/1
  Rate Limit Calculation/4(nz_limit_lo_g) -> Out Bus Element10/1
  In Bus Element7/1 -> Lag Filter/1
  Lag Filter/1 -> Flare Mode/1(flare_Theta_deg), Out Bus Element11/1
  In Bus Element8/1 -> Flare Mode/3(H_radio_ft)
  Flare Mode/1(in_flare) -> Freeze Trim/1(in_flare), Out Bus Element1/1
  Constant/1 -> Manual Switch/2, Manual Switch1/2
  Constant1/1 -> Manual Switch/1, Manual Switch1/1
  Manual Switch/1 -> Flare Mode/4(flare_override_1)
  Manual Switch1/1 -> Flare Mode/5(flare_override_2)
  Abs/1 -> Rate Limiter Dynamic (Variable Ts)/1
  Flare Mode/3(flare_Theta_c_rate_deg_s) -> Out Bus Element13/1, Rate Limiter Dynamic (Variable Ts)/3, Abs/1
  Flare Mode/2(flare_Theta_c_deg) -> Rate Limiter Dynamic (Variable Ts)/2
  Rate Limiter Dynamic (Variable Ts)/1 -> Out Bus Element12/1
  In Bus Element9/1 -> Gain/1
  Gain/1 -> Out Bus Element14/1
  Rate Limiter (Variable Ts)/1 -> Out Bus Element2/1
  In Bus Element10/1 -> Rate Limiter (Variable Ts)/2
  In Bus Element11/1 -> Rate Limiter Dynamic (Variable Ts)/4
  In Bus Element12/1 -> Lag Filter/2
  In Bus Element13/1 -> In Flight/4(time)

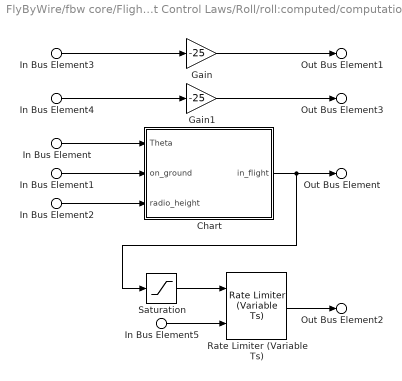
== system FlyByWire/fbw core/Flight Control Laws/Roll/roll:computed/computation ==
  In Bus Element : Inport  PortName=in  Element=sim.data.Theta_deg
  In Bus Element2 : Inport  PortName=in  Element=sim.data.H_radio_ft
  In Bus Element1 : Inport  PortName=in  Element=sim.data_computed.on_ground
  In Bus Element3 : Inport  PortName=in  Element=sim.input.delta_xi_pos
  In Bus Element4 : Inport  PortName=in  Element=sim.input.delta_zeta_pos
  In Bus Element5 : Inport  PortName=in  Element=sim.time.dt
  Chart : Stateflow chart  TreatAsAtomicUnit=on
  Gain : Gain  Gain=-25
  Gain1 : Gain  Gain=-25
  Rate Limiter (Variable Ts) : fbw_library/Rate Limiter (Variable Ts)  up=1/0.5  lo=-1/0.5  InitialCondition=0.0
  Saturation : Saturate  UpperLimit=1  LowerLimit=0
  Out Bus Element1 : Outport  PortName=out  Element=delta_xi_deg
  Out Bus Element3 : Outport  PortName=out  Element=delta_zeta_deg
  Out Bus Element : Outport  PortName=out  Element=in_flight
  Out Bus Element2 : Outport  PortName=out  Element=in_flight_gain
  wires:
  Saturation/1 -> Rate Limiter (Variable Ts)/1
  Rate Limiter (Variable Ts)/1 -> Out Bus Element2/1
  Chart/1(in_flight) -> Out Bus Element/1, Saturation/1
  In Bus Element/1 -> Chart/1(Theta)
  In Bus Element1/1 -> Chart/2(on_ground)
  In Bus Element2/1 -> Chart/3(radio_height)
  In Bus Element3/1 -> Gain/1
  In Bus Element4/1 -> Gain1/1
  Gain/1 -> Out Bus Element1/1
  Gain1/1 -> Out Bus Element3/1
  In Bus Element5/1 -> Rate Limiter (Variable Ts)/2

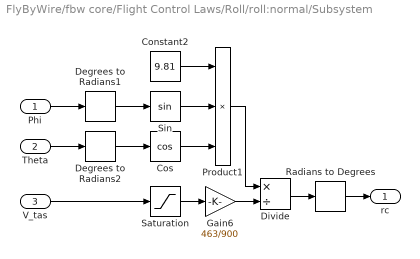
== system FlyByWire/fbw core/Flight Control Laws/Roll/roll:normal/Subsystem ==
  Phi : Inport
  Theta : Inport  Port=2
  V_tas : Inport  Port=3
  Constant2 : Constant  Value=9.81
  Cos : Trigonometry  Operator=cos
  Degrees to Radians1 : simulink_extras/Transformations/Degrees to Radians
  Degrees to Radians2 : simulink_extras/Transformations/Degrees to Radians
  Divide : Product  Inputs=*/
  Gain6 : Gain  Gain=463/900
  Product1 : Product  Inputs=3
  Radians to Degrees : simulink_extras/Transformations/Radians to Degrees
  Saturation : Saturate  UpperLimit=1000  LowerLimit=100
  Sin : Trigonometry
  rc : Outport
  wires:
  Sin/1 -> Product1/2
  Constant2/1 -> Product1/1
  Divide/1 -> Radians to Degrees/1
  Degrees to Radians1/1 -> Sin/1
  Product1/1 -> Divide/1
  V_tas/1 -> Saturation/1
  Gain6/1 -> Divide/2
  Cos/1 -> Product1/3
  Degrees to Radians2/1 -> Cos/1
  Theta/1 -> Degrees to Radians2/1
  Phi/1 -> Degrees to Radians1/1
  Radians to Degrees/1 -> rc/1
  Saturation/1 -> Gain6/1

== system FlyByWire/fbw core/Flight Control Laws/Pitch/pitch/law_normal/C* Calculation ==
  nz (g) : Inport
  qk (°/s) : Inport  Port=2
  Vtas (kn) : Inport  Port=3
  1-D Lookup Table : Lookup_n-D  NumberOfTableDimensions=1  BreakpointsForDimension1=[0 100 210 350 500]  Table=[12.4 12.4 12.4 12.4 12.4]  InternalRulePriority=Speed  RndMeth=Simplest  InputSameDT=on
  Degrees to Radians : simulink_extras/Transformations/Degrees to Radians
  Product : Product
  Sum : Sum  Inputs=|++
  C* (g) : Outport
  wires:
  1-D Lookup Table/1 -> Product/2
  Degrees to Radians/1 -> Product/1
  Product/1 -> Sum/2
  qk (°/s)/1 -> Degrees to Radians/1
  nz (g)/1 -> Sum/1
  Sum/1 -> C* (g)/1
  Vtas (kn)/1 -> 1-D Lookup Table/1

== system FlyByWire/fbw core/Flight Control Laws/Pitch/pitch/law_normal/Curve Compensation ==
  Theta : Inport
  Phi : Inport  Port=2
  Cos : Trigonometry  Operator=cos
  Cos1 : Trigonometry  Operator=cos
  Degrees to Radians : simulink_extras/Transformations/Degrees to Radians
  Degrees to Radians1 : simulink_extras/Transformations/Degrees to Radians
  Divide : Product  Inputs=*/
  Saturation : Saturate  UpperLimit=33  LowerLimit=-33
  Factor : Outport
  wires:
  Degrees to Radians1/1 -> Cos1/1
  Degrees to Radians/1 -> Cos/1
  Cos1/1 -> Divide/2
  Cos/1 -> Divide/1
  Theta/1 -> Degrees to Radians/1
  Phi/1 -> Saturation/1
  Divide/1 -> Factor/1
  Saturation/1 -> Degrees to Radians1/1

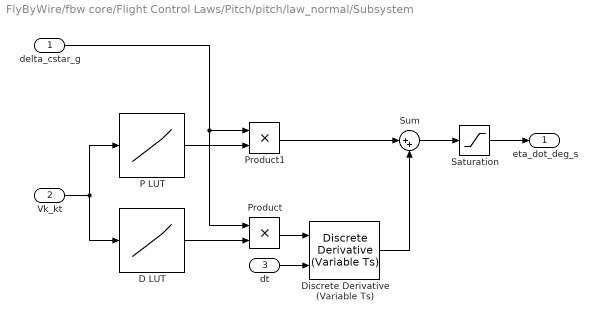
== system FlyByWire/fbw core/Flight Control Laws/Pitch/pitch/law_normal/Subsystem ==
  delta_cstar_g : Inport
  Vk_kt : Inport  Port=2
  dt : Inport  Port=3
  D LUT : Lookup_n-D  NumberOfTableDimensions=1  BreakpointsForDimension1=[0 350]  Table=[1.5 6]  InternalRulePriority=Speed  RndMeth=Simplest  InputSameDT=on
  Discrete Derivative (Variable Ts) : fbw_library/Discrete Derivative (Variable Ts)  Gain=1.0  InitialCondition=0.0
  P LUT : Lookup_n-D  NumberOfTableDimensions=1  BreakpointsForDimension1=[0 350]  Table=[13.5 13.5]  InternalRulePriority=Speed  RndMeth=Simplest  InputSameDT=on
  Product : Product
  Product1 : Product
  Saturation : Saturate  UpperLimit=17  LowerLimit=-30
  Sum : Sum  Inputs=|++
  eta_dot_deg_s : Outport
  wires:
  Vk_kt/1 -> D LUT/1, P LUT/1
  P LUT/1 -> Product1/2
  Sum/1 -> Saturation/1
  D LUT/1 -> Product/2
  Product/1 -> Discrete Derivative (Variable Ts)/1
  delta_cstar_g/1 -> Product1/1, Product/1
  Product1/1 -> Sum/1
  Discrete Derivative (Variable Ts)/1 -> Sum/2
  Saturation/1 -> eta_dot_deg_s/1
  dt/1 -> Discrete Derivative (Variable Ts)/2

== stateflow chart FlyByWire/fbw core/Flight Control Laws/Pitch/pitch:computed/computation/In Flight ==
  state Ground
    in_flight = 0;
  state Flight
    in_flight = 1;
  state FlightToGroundTransition
  (junction 40) -> (junction 41) : [(on_ground == 0 & Theta_deg > 8) | H_radio_ft > 400]
      | {on_ground_time = 0}
  Ground -> (junction 40)
  (junction 41) -> Flight
  (default) -> Ground
  (junction 56) -> Flight
  FlightToGroundTransition -> (junction 56) [order 2] : [on_ground == 0 | Theta_deg >= 2.5]
      | {on_ground_time = 0}
  (junction 46) -> Ground
  Flight -> (junction 48) : [on_ground == 1 & Theta_deg < 2.5]
      | {on_ground_time = time}
  (junction 48) -> FlightToGroundTransition
  FlightToGroundTransition -> (junction 46) [order 1] : [(time - on_ground_time) >= 5]
  data: Theta_deg input; H_radio_ft input; in_flight output [0..1]; on_ground input [0..1]; time input [0..]; on_ground_time local

== matlab function FlyByWire/fbw core/Flight Control Laws/Pitch/pitch:vote/Voter ==
  data: input input; vote output
function vote = Voter(input)
vote = median(input);

== stateflow chart FlyByWire/fbw core/Flight Control Laws/Roll/roll:computed/computation/Chart ==
  state GroundMode
    in_flight = 0;
  state FlightMode
    in_flight = 1;
  GroundMode -> FlightMode : [(on_ground == 0 & Theta > 8) | radio_height > 400]
  (default) -> GroundMode
  FlightMode -> GroundMode : [on_ground == 1]
  data: Theta input; on_ground input [0..1]; in_flight output [0..1]; radio_height input

== stateflow chart FlyByWire/fbw core/Flight Control Laws/Pitch/pitch:computed/computation/Rate Limit Calculation ==
  state flight_clean
    eta_trim_deg_rate_limit_up_deg_s = 0.3;
    eta_trim_deg_rate_limit_lo_deg_s = -0.3;
    nz_limit_up_g = 2.5;
    nz_limit_lo_g = -1;
  state ground
    eta_trim_deg_rate_limit_up_deg_s = 0.7;
    eta_trim_deg_rate_limit_lo_deg_s = -0.7;
    nz_limit_up_g = 2;
    nz_limit_lo_g = 0;
  state flight_flaps
    eta_trim_deg_rate_limit_up_deg_s = 0.7;
    eta_trim_deg_rate_limit_lo_deg_s = -0.7;
    nz_limit_up_g = 2;
    nz_limit_lo_g = 0;
  ground -> flight_clean [order 1] : [in_flight & ~flaps_handle_index]
  (default) -> ground
  flight_clean -> ground [order 2] : [~in_flight & ~flaps_handle_index]
  ground -> flight_flaps [order 2] : [in_flight & flaps_handle_index]
  flight_flaps -> flight_clean [order 1] : [~flaps_handle_index]
  flight_clean -> flight_flaps [order 1] : [flaps_handle_index]
  flight_flaps -> ground [order 2] : [~in_flight]
  data: in_flight input [0..1]; flaps_handle_index input [0..4]; eta_trim_deg_rate_limit_up_deg_s output; eta_trim_deg_rate_limit_lo_deg_s output; nz_limit_up_g output; nz_limit_lo_g output

== stateflow chart FlyByWire/fbw core/Flight Control Laws/Pitch/pitch:computed/computation/Manual Trim ==
  state automatic
    eta_trim_deg_reset = false;
    eta_trim_deg_reset_deg = eta_trim_deg;
    eta_trim_deg_should_write = true;
  state manual
    eta_trim_deg_reset = true;
    eta_trim_deg_reset_deg = eta_trim_deg;
    eta_trim_deg_should_write = false;
  state reset
    eta_trim_deg_reset = true;
    eta_trim_deg_reset_deg = 0;
    eta_trim_deg_should_write = true;
  manual -> automatic : [in_flight]
  (default) -> manual
  reset -> manual : [~in_flight & eta_trim_deg == 0]
  automatic -> reset : [~in_flight]
  data: eta_trim_deg_should_write output [0..1]; eta_trim_deg_reset output [0..1]; in_flight input [0..1]; eta_trim_deg input; eta_trim_deg_reset_deg output

== stateflow chart FlyByWire/fbw core/Flight Control Laws/Pitch/pitch:computed/computation/Freeze Trim ==
  state running
    eta_trim_deg_should_freeze = false;
  state frozen
    eta_trim_deg_should_freeze = true;
  running -> frozen : [in_flare | nz_g >= 1.25 | nz_g <= 0.5 | abs(Phi_deg) > 30.0]
  (default) -> running
  frozen -> running : [~in_flare & nz_g < 1.25 & nz_g > 0.5 & abs(Phi_deg) <= 30.0]
  data: in_flare input [0..1]; nz_g input; eta_trim_deg_should_freeze output [0..1]; Phi_deg input

== stateflow chart FlyByWire/fbw core/Data Computation/Calculation/Chart ==
  state OnGround
    on_ground = 1;
  state InAir
    on_ground = 0;
  OnGround -> InAir : [gear_strut_compression_1 == 0 & gear_strut_compression_2 == 0]
  (default) -> OnGround
  InAir -> OnGround : [gear_strut_compression_1 > 0.1 | gear_strut_compression_2 > 0.1]
  data: on_ground output [0..1]; gear_strut_compression_1 input [0..1]; gear_strut_compression_2 input [0..1]

== stateflow chart FlyByWire/fbw core/Flight Control Laws/Pitch/pitch:computed/computation/Flare Mode ==
  state Flight_High
    in_flare = 0;
    flare_Theta_c_deg = flare_Theta_deg;
    flare_Theta_c_rate_deg_s = -3;
  state Ground
    in_flare = 0;
    flare_Theta_c_deg = flare_Theta_deg;
    flare_Theta_c_rate_deg_s = -3;
  state Flight_Low
    in_flare = 0;
    flare_Theta_c_deg = flare_Theta_deg;
    flare_Theta_c_rate_deg_s = -3;
  state Flare_Reduce_Theta_c
    in_flare = 1;
    flare_Theta_c_deg = -2;
  state Flare_Set_Rate
    in_flare = 1;
  state Flare_Store_Theta_c_deg
    in_flare = 1;
  (junction 40) -> (junction 41) : [in_flight == 1]
  Ground -> (junction 40)
  (junction 41) -> Flight_Low
  (default) -> Ground
  Flight_Low -> Flight_High : [H_radio_ft > 50]
  (junction 57) -> Flight_Low : [H_radio_ft > 50 & flare_override_1 == 0]
  Flare_Reduce_Theta_c -> Ground [order 1] : [in_flight == 0]
  Flight_High -> (junction 44) : [H_radio_ft <= 50 | flare_override_1 == 1]
  (junction 66) -> (junction 57)
  (junction 64) -> (junction 57)
  Flare_Reduce_Theta_c -> (junction 66) [order 2]
  Flare_Set_Rate -> (junction 57) [order 2]
  Flare_Store_Theta_c_deg -> (junction 64) [order 1]
  (junction 44) -> Flare_Store_Theta_c_deg : { flare_Theta_c_deg = flare_Theta_deg }
  Flare_Store_Theta_c_deg -> Flare_Set_Rate [order 2] : { flare_Theta_c_rate_deg_s = -1 * (flare_Theta_deg + 2) / 8 }
  Flare_Set_Rate -> Flare_Reduce_Theta_c [order 1] : [H_radio_ft <= 30 | flare_override_2 == 1]
  data: flare_Theta_deg input; in_flight input [0..1]; H_radio_ft input; in_flare output [0..1]; flare_Theta_c_deg output; flare_Theta_c_rate_deg_s output; flare_override_1 input; flare_override_2 input
